simulink model "Sys_iden_block"  (R2026a)
settings: Solver=VariableStepAuto
libraries: arduinolib x2
settings Model: Creator=kanis  LastModifiedBy=kanis

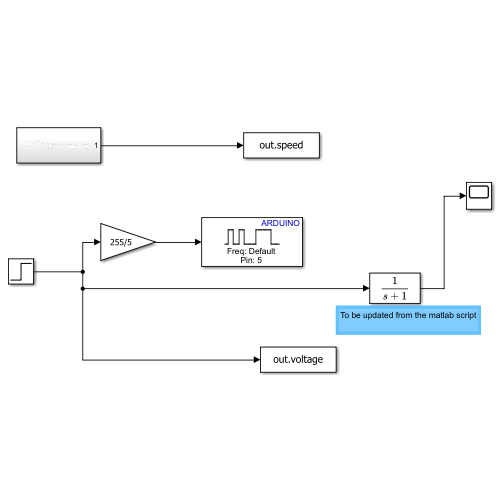
[thumbnail: Simulink's stored preview of the top-level diagram]
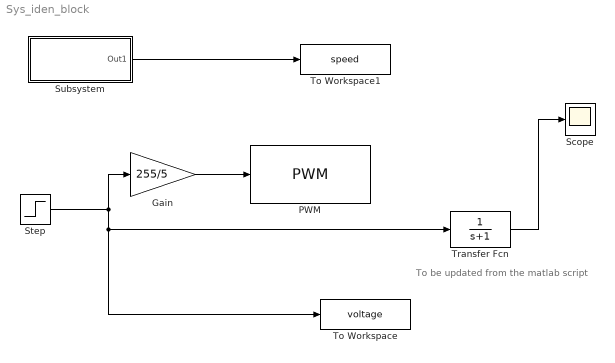
== system Sys_iden_block ==
  note: To be updated from the matlab script
  Gain : Gain  Gain=255/5
  PWM : arduinolib/PWM  pinNumber=5  frequencyType=Default  desiredFrequency=490.2  achievableFrequency=490.2
  Scope : Scope
  Step : Step  Time=0  FinalValue=5  SampleTime=0
  Subsystem : Subsystem
  To Workspace : ToWorkspace  VariableName=voltage  SaveFormat=Timeseries  SampleTime=-1
  To Workspace1 : ToWorkspace  VariableName=speed  SaveFormat=Timeseries  SampleTime=-1
  Transfer Fcn : TransferFcn  Denominator=[1 1]
  wires:
  Step/1 -> To Workspace/1, Transfer Fcn/1, Gain/1
  Gain/1 -> PWM/1
  Subsystem/1(Out1) -> To Workspace1/1
  Transfer Fcn/1 -> Scope/1

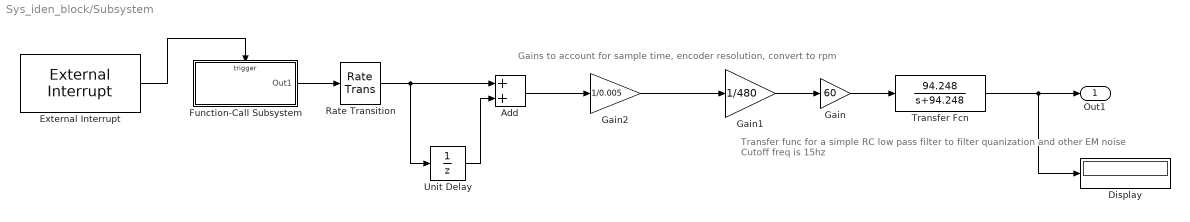
== system Sys_iden_block/Subsystem ==
  note: Gains to account for sample time, encoder resolution, convert to rpm
  note: Transfer func for a simple RC low pass filter to filter quanization and other EM noise
      | Cutoff freq is 15hz
  Add : Sum
  Display : Display
  External Interrupt : arduinolib/External Interrupt  Pin=2  PullUp=off  Mode=RISING  InterruptSimulationInput=off
  Function-Call Subsystem : Subsystem  TreatAsAtomicUnit=on
  Gain : Gain  Gain=60
  Gain1 : Gain  Gain=1/480
  Gain2 : Gain  Gain=1/0.005
  Rate Transition : RateTransition
  Transfer Fcn : TransferFcn  Numerator=94.248  Denominator=[1, 94.248]
  Unit Delay : UnitDelay  SampleTime=-1
  Out1 : Outport
  wires:
  Gain2/1 -> Gain1/1
  Gain1/1 -> Gain/1
  Gain/1 -> Transfer Fcn/1
  Transfer Fcn/1 -> Display/1, Out1/1
  Add/1 -> Gain2/1
  Rate Transition/1 -> Unit Delay/1, Add/1
  Unit Delay/1 -> Add/2
  Function-Call Subsystem/1(Out1) -> Rate Transition/1
  External Interrupt/1 -> Function-Call Subsystem/Trigger

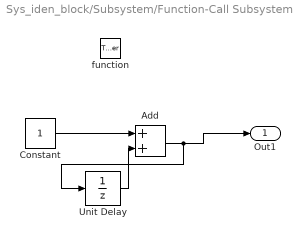
== system Sys_iden_block/Subsystem/Function-Call Subsystem ==
  function : TriggerPort  TriggerType=function-call  VariantControl=(inherit)
  Add : Sum
  Constant : Constant
  Unit Delay : UnitDelay  SampleTime=-1
  Out1 : Outport
  wires:
  Constant/1 -> Add/1
  Add/1 -> Unit Delay/1, Out1/1
  Unit Delay/1 -> Add/2
